simulink model "InvertedPendulumRobot_ControllerDesignLab"  (R2015b)
settings: Solver=FixedStepAuto  StartTime=0.0  StopTime=inf  RelTol=1e-3
libraries: arduinolib x10, simulink x2, aerolibtransform2 x1
settings Model: SimulationMode=external  ExtModeTrigDuration=2  Creator=james_000  LastModifiedBy=james_000
settings OptimizationCC: OptimizeModelRefInitCode=on  LifeSpan=1  MaxStackSize=64
settings DebuggingCC: InheritedTsInSrcMsg=none
settings HardwareCC: ProdBitPerInt=16  ProdBitPerPointer=16  ProdLargestAtomicFloat=None  ProdWordSize=8  ProdHWDeviceType=Atmel->AVR
settings RTWCC: SystemTargetFile=ert.tlc  TemplateMakefile=ert_default_tmf  Description=Embedded Coder  Toolchain=Arduino AVR v1.6.1  BuildConfiguration=Faster Runs  PortableWordSizes=on
settings CodeAppCC: IgnoreCustomStorageClasses=off
settings ERTTargetCC: SupportContinuousTime=on  SupportVariableSizeSignals=on  ExtMode=on  ExtModeMexArgs=0 7 115200

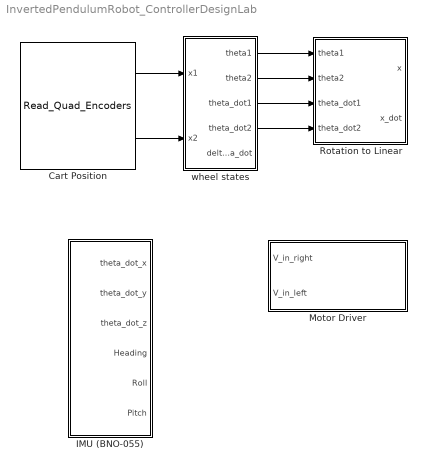
== system InvertedPendulumRobot_ControllerDesignLab ==
  Cart Position : S-Function  InitFcn=try, set_param(gcb,'FunctionName','Read_Quad_Encoders'), end  FunctionName=Read_Quad_Encoders  Parameters=uint8([0 1]),uint8([2 3]),uint8([7 8])  SFunctionModules=Read_Quad_Encoders_wrapper  SFunctionDeploymentMode=off  EnableBusSupport=off  mask(S-Function Builder){}
      mask help: Simulink:masks:SFunctionBuilder_MD
      mask init:
      | val = [[.9  0.75 0.75 1 1 .9 .9 1]',[1 1 0.75 0.75 .9 .9 1 .9]'];try , sys = get_param(gcb,'SfunBuilderFcnName');if isempty(sys), sys = get_param(gcb,'FunctionName'); end,catch, sys = get_param(gcb,'FunctionName'); end
      settings: CopyFcn=set_param(gcbh,'LinkStatus','none')  PreSaveFcn=try, set_param(gcb,'FunctionName','Read_Quad_Encoders'), end  OpenFcn=sfunctionwizard(gcbh)
      mask Display: plot(val(:,1),val(:,2)),disp(sys), port_label('output',1,'x1'), port_label('output',2,'x2')
  IMU (BNO-055) : Subsystem
  Motor Driver : Subsystem
  Rotation to Linear : Subsystem
  wheel states : Subsystem
  wires:
  Cart Position/1 -> wheel states/1(x1)
  Cart Position/2 -> wheel states/2(x2)
  wheel states/4(theta_dot2) -> Rotation to Linear/4(theta_dot2)
  wheel states/3(theta_dot1) -> Rotation to Linear/3(theta_dot1)
  wheel states/2(theta2) -> Rotation to Linear/2(theta2)
  wheel states/1(theta1) -> Rotation to Linear/1(theta1)

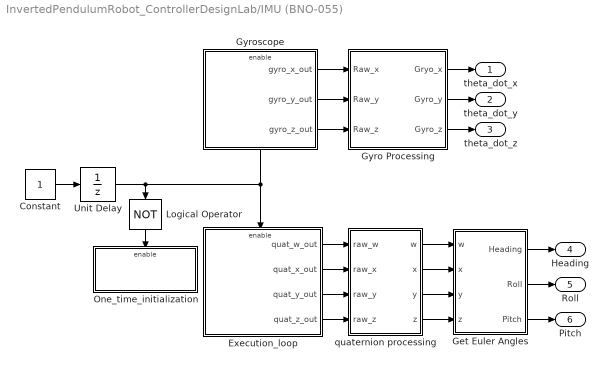
== system InvertedPendulumRobot_ControllerDesignLab/IMU (BNO-055) ==
  Constant : Constant  OutDataTypeStr=boolean  SampleTime=0.02
  Execution_loop : Subsystem  TreatAsAtomicUnit=on
  Get Euler Angles : Subsystem
  Gyro Processing : Subsystem
  Gyroscope : Subsystem  TreatAsAtomicUnit=on
  Logical Operator : Logic  Operator=NOT  AllPortsSameDT=off  OutDataTypeStr=boolean
  One_time_initialization : Subsystem  TreatAsAtomicUnit=on
  Unit Delay : UnitDelay  SampleTime=0.02
  quaternion processing : Subsystem
  theta_dot_x : Outport
  theta_dot_y : Outport  Port=2
  theta_dot_z : Outport  Port=3
  Heading : Outport  Port=4
  Roll : Outport  Port=5
  Pitch : Outport  Port=6
  wires:
  Constant/1 -> Unit Delay/1
  Logical Operator/1 -> One_time_initialization/Enable
  Unit Delay/1 -> Gyroscope/Enable, Execution_loop/Enable, Logical Operator/1
  Gyroscope/1(gyro_x_out) -> Gyro Processing/1(Raw_x)
  Gyroscope/2(gyro_y_out) -> Gyro Processing/2(Raw_y)
  Gyroscope/3(gyro_z_out) -> Gyro Processing/3(Raw_z)
  Gyro Processing/1(Gryo_x) -> theta_dot_x/1
  Gyro Processing/2(Gyro_y) -> theta_dot_y/1
  Gyro Processing/3(Gyro_z) -> theta_dot_z/1
  Get Euler Angles/1(Heading) -> Heading/1
  Execution_loop/1(quat_w_out) -> quaternion processing/1(raw_w)
  Execution_loop/2(quat_x_out) -> quaternion processing/2(raw_x)
  Execution_loop/3(quat_y_out) -> quaternion processing/3(raw_y)
  Execution_loop/4(quat_z_out) -> quaternion processing/4(raw_z)
  quaternion processing/1(w) -> Get Euler Angles/1(w)
  quaternion processing/2(x) -> Get Euler Angles/2(x)
  quaternion processing/3(y) -> Get Euler Angles/3(y)
  quaternion processing/4(z) -> Get Euler Angles/4(z)
  Get Euler Angles/2(Roll) -> Roll/1
  Get Euler Angles/3(Pitch) -> Pitch/1

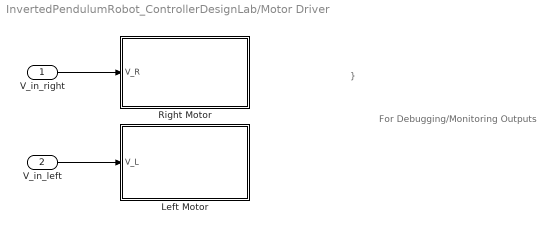
== system InvertedPendulumRobot_ControllerDesignLab/Motor Driver ==
  note: }
  note: For Debugging/Monitoring Outputs
  V_in_right : Inport
  V_in_left : Inport  Port=2
  Left Motor : Subsystem
  Right Motor : Subsystem
  wires:
  V_in_left/1 -> Left Motor/1(V_L)
  V_in_right/1 -> Right Motor/1(V_R)

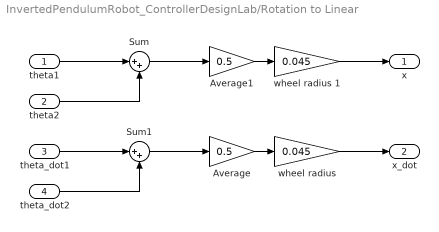
== system InvertedPendulumRobot_ControllerDesignLab/Rotation to Linear ==
  theta1 : Inport
  theta2 : Inport  Port=2
  theta_dot1 : Inport  Port=3
  theta_dot2 : Inport  Port=4
  Average : Gain  Gain=0.5
  Average1 : Gain  Gain=0.5
  Sum : Sum  Inputs=|++
  Sum1 : Sum  Inputs=|++
  wheel radius : Gain  Gain=0.045
  wheel radius 1 : Gain  Gain=0.045
  x : Outport
  x_dot : Outport  Port=2
  wires:
  theta2/1 -> Sum/2
  theta1/1 -> Sum/1
  Sum/1 -> Average1/1
  Average1/1 -> wheel radius 1/1
  theta_dot2/1 -> Sum1/2
  theta_dot1/1 -> Sum1/1
  Sum1/1 -> Average/1
  Average/1 -> wheel radius/1
  wheel radius 1/1 -> x/1
  wheel radius/1 -> x_dot/1

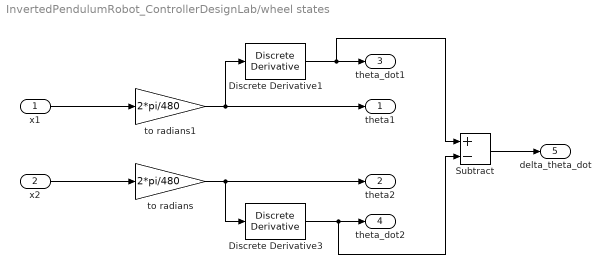
== system InvertedPendulumRobot_ControllerDesignLab/wheel states ==
  x1 : Inport
  x2 : Inport  Port=2
  Discrete Derivative1 : simulink/Discrete/Discrete Derivative  gainval=1.0  ICPrevScaledInput=0.0  InputProcessing=Inherited  OutMin=[]  OutMax=[]  OutDataType=fixdt(1, 16)  OutScaling=2^-10  DoSatur=off
  Discrete Derivative3 : simulink/Discrete/Discrete Derivative  gainval=1.0  ICPrevScaledInput=0.0  InputProcessing=Inherited  OutMin=[]  OutMax=[]  OutDataType=fixdt(1, 16)  OutScaling=2^-10  DoSatur=off
  Subtract : Sum  Inputs=+-
  to radians : Gain  Gain=2*pi/480
  to radians1 : Gain  Gain=2*pi/480
  theta1 : Outport
  theta2 : Outport  Port=2
  theta_dot1 : Outport  Port=3
  theta_dot2 : Outport  Port=4
  delta_theta_dot : Outport  Port=5
  wires:
  x2/1 -> to radians/1
  x1/1 -> to radians1/1
  to radians1/1 -> Discrete Derivative1/1, theta1/1
  Discrete Derivative1/1 -> Subtract/1, theta_dot1/1
  to radians/1 -> Discrete Derivative3/1, theta2/1
  Discrete Derivative3/1 -> Subtract/2, theta_dot2/1
  Subtract/1 -> delta_theta_dot/1

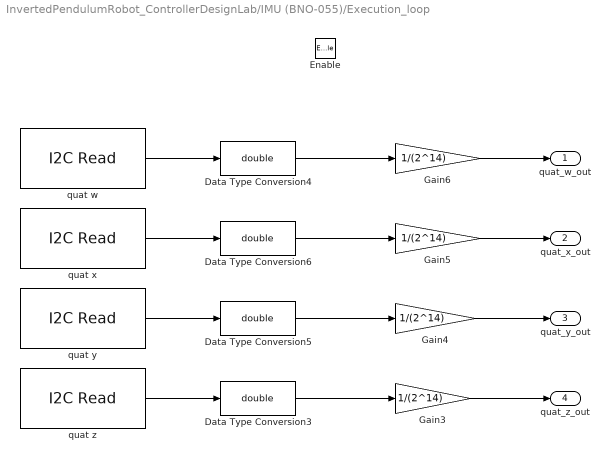
== system InvertedPendulumRobot_ControllerDesignLab/IMU (BNO-055)/Execution_loop ==
  Enable : EnablePort
  Data Type Conversion{3..6} (4 alike) : DataTypeConversion  OutDataTypeStr=double  ConvertRealWorld=Stored Integer (SI)
  Gain{3..6} (4 alike) : Gain  Gain=1/(2^14)
  quat w : arduinolib/I2C Read  SlaveAddress_=hex2dec( '28' )  RegisterAddressEnable=on  RegisterAddress_=hex2dec( '20' )  Datatype=uint16  ByteOrder=Little Endian  Datalength_=1  SampleTime_=0.02  blockPlatform=arduino
  quat x : arduinolib/I2C Read  SlaveAddress_=hex2dec( '28' )  RegisterAddressEnable=on  RegisterAddress_=hex2dec( '22' )  Datatype=uint16  ByteOrder=Little Endian  Datalength_=1  SampleTime_=0.02  blockPlatform=arduino
  quat y : arduinolib/I2C Read  SlaveAddress_=hex2dec( '28' )  RegisterAddressEnable=on  RegisterAddress_=hex2dec( '24' )  Datatype=uint16  ByteOrder=Little Endian  Datalength_=1  SampleTime_=0.02  blockPlatform=arduino
  quat z : arduinolib/I2C Read  SlaveAddress_=hex2dec( '28' )  RegisterAddressEnable=on  RegisterAddress_=hex2dec( '26' )  Datatype=uint16  ByteOrder=Little Endian  Datalength_=1  SampleTime_=0.02  blockPlatform=arduino
  quat_w_out : Outport
  quat_x_out : Outport  Port=2
  quat_y_out : Outport  Port=3
  quat_z_out : Outport  Port=4
  wires:
  quat x/1 -> Data Type Conversion6/1
  quat w/1 -> Data Type Conversion4/1
  quat y/1 -> Data Type Conversion5/1
  quat z/1 -> Data Type Conversion3/1
  Data Type Conversion4/1 -> Gain6/1
  Data Type Conversion6/1 -> Gain5/1
  Data Type Conversion5/1 -> Gain4/1
  Data Type Conversion3/1 -> Gain3/1
  Gain6/1 -> quat_w_out/1
  Gain5/1 -> quat_x_out/1
  Gain4/1 -> quat_y_out/1
  Gain3/1 -> quat_z_out/1

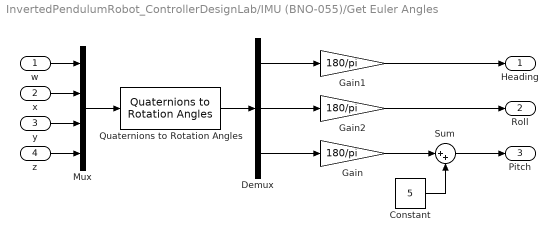
== system InvertedPendulumRobot_ControllerDesignLab/IMU (BNO-055)/Get Euler Angles ==
  w : Inport
  x : Inport  Port=2
  y : Inport  Port=3
  z : Inport  Port=4
  Constant : Constant  Value=5
  Demux : Demux  Outputs=3
  Gain : Gain  Gain=180/pi
  Gain1 : Gain  Gain=180/pi
  Gain2 : Gain  Gain=180/pi
  Mux : Mux
  Quaternions to Rotation Angles : aerolibtransform2/Quaternions to Rotation Angles  rotationOrder=ZYX
  Sum : Sum  Inputs=|++
  Heading : Outport
  Roll : Outport  Port=2
  Pitch : Outport  Port=3
  wires:
  Mux/1 -> Quaternions to Rotation Angles/1
  Quaternions to Rotation Angles/1 -> Demux/1
  Demux/2 -> Gain2/1
  Demux/1 -> Gain1/1
  w/1 -> Mux/1
  x/1 -> Mux/2
  y/1 -> Mux/3
  z/1 -> Mux/4
  Demux/3 -> Gain/1
  Sum/1 -> Pitch/1
  Constant/1 -> Sum/2
  Gain/1 -> Sum/1
  Gain2/1 -> Roll/1
  Gain1/1 -> Heading/1

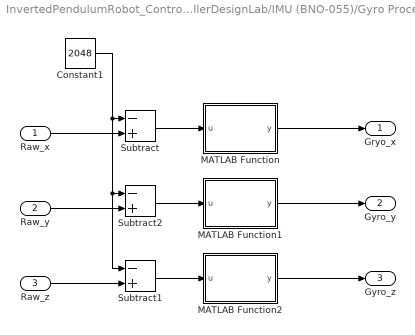
== system InvertedPendulumRobot_ControllerDesignLab/IMU (BNO-055)/Gyro Processing ==
  Raw_x : Inport
  Raw_y : Inport  Port=2
  Raw_z : Inport  Port=3
  Constant1 : Constant  Value=2048  OutDataTypeStr=double
  MATLAB Function : MATLAB Function  TreatAsAtomicUnit=on
  MATLAB Function1 : MATLAB Function  TreatAsAtomicUnit=on
  MATLAB Function2 : MATLAB Function  TreatAsAtomicUnit=on
  Subtract : Sum  Inputs=-+  OutDataTypeStr=double
  Subtract1 : Sum  Inputs=-+  OutDataTypeStr=double
  Subtract2 : Sum  Inputs=-+  OutDataTypeStr=double
  Gryo_x : Outport
  Gyro_y : Outport  Port=2
  Gyro_z : Outport  Port=3
  wires:
  Raw_x/1 -> Subtract/2
  Raw_z/1 -> Subtract1/2
  Raw_y/1 -> Subtract2/2
  MATLAB Function1/1(y) -> Gyro_y/1
  Subtract/1 -> MATLAB Function/1(u)
  Subtract2/1 -> MATLAB Function1/1(u)
  Subtract1/1 -> MATLAB Function2/1(u)
  Constant1/1 -> Subtract/1, Subtract2/1, Subtract1/1
  MATLAB Function/1(y) -> Gryo_x/1
  MATLAB Function2/1(y) -> Gyro_z/1

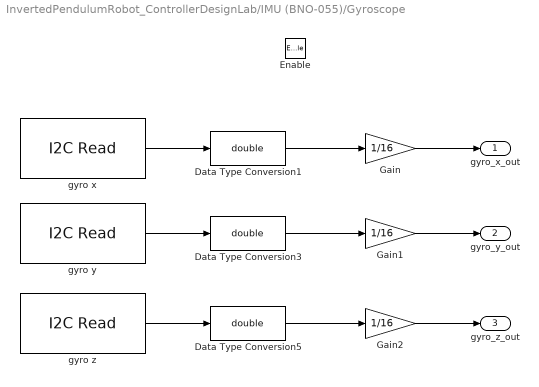
== system InvertedPendulumRobot_ControllerDesignLab/IMU (BNO-055)/Gyroscope ==
  Enable : EnablePort
  Data Type Conversion1 : DataTypeConversion  OutDataTypeStr=double
  Data Type Conversion3 : DataTypeConversion  OutDataTypeStr=double
  Data Type Conversion5 : DataTypeConversion  OutDataTypeStr=double
  Gain : Gain  Gain=1/16  OutDataTypeStr=Inherit: Same as input
  Gain1 : Gain  Gain=1/16  OutDataTypeStr=Inherit: Same as input
  Gain2 : Gain  Gain=1/16  OutDataTypeStr=Inherit: Same as input
  gyro x : arduinolib/I2C Read  SlaveAddress_=hex2dec( '28' )  RegisterAddressEnable=on  RegisterAddress_=hex2dec( '14' )  Datatype=uint16  ByteOrder=Little Endian  Datalength_=1  SampleTime_=0.02  blockPlatform=arduino
  gyro y : arduinolib/I2C Read  SlaveAddress_=hex2dec( '28' )  RegisterAddressEnable=on  RegisterAddress_=hex2dec( '16' )  Datatype=uint16  ByteOrder=Little Endian  Datalength_=1  SampleTime_=0.02  blockPlatform=arduino
  gyro z : arduinolib/I2C Read  SlaveAddress_=hex2dec( '28' )  RegisterAddressEnable=on  RegisterAddress_=hex2dec( '18' )  Datatype=uint16  ByteOrder=Little Endian  Datalength_=1  SampleTime_=0.02  blockPlatform=arduino
  gyro_x_out : Outport
  gyro_y_out : Outport  Port=2
  gyro_z_out : Outport  Port=3
  wires:
  Gain/1 -> gyro_x_out/1
  Gain1/1 -> gyro_y_out/1
  Gain2/1 -> gyro_z_out/1
  gyro x/1 -> Data Type Conversion1/1
  Data Type Conversion3/1 -> Gain1/1
  Data Type Conversion5/1 -> Gain2/1
  gyro y/1 -> Data Type Conversion3/1
  gyro z/1 -> Data Type Conversion5/1
  Data Type Conversion1/1 -> Gain/1

== system InvertedPendulumRobot_ControllerDesignLab/IMU (BNO-055)/One_time_initialization ==
  Enable : EnablePort
  Constant2 : Constant  Value=8  OutDataTypeStr=uint8
  I2C Write2 : arduinolib/I2C Write  Priority=1  SlaveAddress_=hex2dec( '28' )  RegisterAddressEnable=on  RegisterAddress_=hex2dec( '3D' )  Datatype=uint8  ByteOrder=Big Endian  blockPlatform=arduino
      settings: AttributesFormatString=Priority=%<Priority>
  wires:
  Constant2/1 -> I2C Write2/1

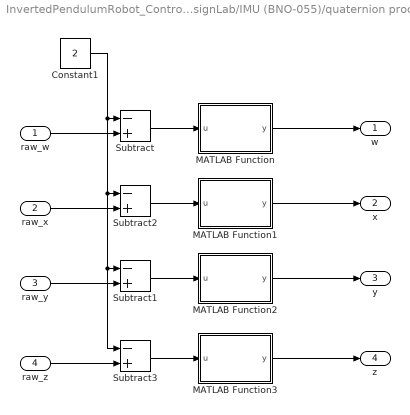
== system InvertedPendulumRobot_ControllerDesignLab/IMU (BNO-055)/quaternion processing ==
  raw_w : Inport
  raw_x : Inport  Port=2
  raw_y : Inport  Port=3
  raw_z : Inport  Port=4
  Constant1 : Constant  Value=2  OutDataTypeStr=double
  MATLAB Function : MATLAB Function  TreatAsAtomicUnit=on
  MATLAB Function1 : MATLAB Function  TreatAsAtomicUnit=on
  MATLAB Function2 : MATLAB Function  TreatAsAtomicUnit=on
  MATLAB Function3 : MATLAB Function  TreatAsAtomicUnit=on
  Subtract{,1..3} (4 alike) : Sum  Inputs=-+  OutDataTypeStr=double
  w : Outport
  x : Outport  Port=2
  y : Outport  Port=3
  z : Outport  Port=4
  wires:
  raw_x/1 -> Subtract2/2
  Subtract2/1 -> MATLAB Function1/1(u)
  Subtract1/1 -> MATLAB Function2/1(u)
  Subtract/1 -> MATLAB Function/1(u)
  raw_w/1 -> Subtract/2
  raw_y/1 -> Subtract1/2
  MATLAB Function1/1(y) -> x/1
  Constant1/1 -> Subtract/1, Subtract2/1, Subtract3/1, Subtract1/1
  MATLAB Function2/1(y) -> y/1
  MATLAB Function/1(y) -> w/1
  Subtract3/1 -> MATLAB Function3/1(u)
  raw_z/1 -> Subtract3/2
  MATLAB Function3/1(y) -> z/1

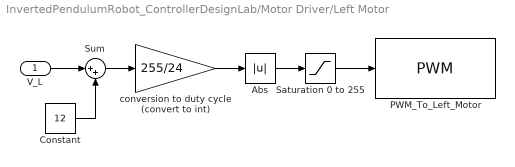
== system InvertedPendulumRobot_ControllerDesignLab/Motor Driver/Left Motor ==
  V_L : Inport
  Abs : Abs
  Constant : Constant  Value=12
  PWM_To_Left_Motor : arduinolib/PWM  pinNumber=5  blockPlatform=arduino
  Saturation 0 to 255 : Saturate  UpperLimit=255  LowerLimit=0
  Sum : Sum  Inputs=|++
  conversion to duty cycle (convert to int) : Gain  Gain=255/24  OutDataTypeStr=int16
  wires:
  Saturation 0 to 255/1 -> PWM_To_Left_Motor/1
  conversion to duty cycle (convert to int)/1 -> Abs/1
  Abs/1 -> Saturation 0 to 255/1
  V_L/1 -> Sum/1
  Sum/1 -> conversion to duty cycle (convert to int)/1
  Constant/1 -> Sum/2

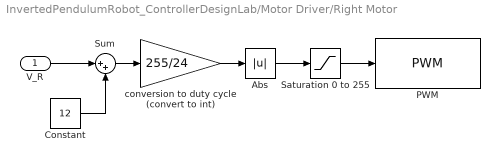
== system InvertedPendulumRobot_ControllerDesignLab/Motor Driver/Right Motor ==
  V_R : Inport
  Abs : Abs
  Constant : Constant  Value=12
  PWM : arduinolib/PWM  pinNumber=3  blockPlatform=arduino
  Saturation 0 to 255 : Saturate  UpperLimit=255  LowerLimit=0
  Sum : Sum  Inputs=|++
  conversion to duty cycle (convert to int) : Gain  Gain=255/24  OutDataTypeStr=int16
  wires:
  Abs/1 -> Saturation 0 to 255/1
  Saturation 0 to 255/1 -> PWM/1
  conversion to duty cycle (convert to int)/1 -> Abs/1
  V_R/1 -> Sum/1
  Sum/1 -> conversion to duty cycle (convert to int)/1
  Constant/1 -> Sum/2

== matlab function InvertedPendulumRobot_ControllerDesignLab/IMU (BNO-055)/Gyro Processing/MATLAB Function1 ==
  data: u input; y output
function y = fcn(u)
%#codegen
if u>1000
    u=u-2048;
elseif u<1000
    u=u+2048;
else
    u=u;
end
y = u;

== matlab function InvertedPendulumRobot_ControllerDesignLab/IMU (BNO-055)/Gyro Processing/MATLAB Function ==
  data: u input; y output
function y = fcn(u)
%#codegen
if u>1000
    u=u-2048;
elseif u<1000
    u=u+2048;
else
    u=u;
end
y = u;

== matlab function InvertedPendulumRobot_ControllerDesignLab/IMU (BNO-055)/Gyro Processing/MATLAB Function2 ==
  data: u input; y output
function y = fcn(u)
%#codegen
if u>1000
    u=u-2048;
elseif u<1000
    u=u+2048;
else
    u=u;
end
y = u;

== matlab function InvertedPendulumRobot_ControllerDesignLab/IMU (BNO-055)/quaternion processing/MATLAB Function ==
  data: u input; y output
function y = fcn(u)
%#codegen
if u>1
    u=u-2;
elseif u<-1
    u=u+2;
end
y = u;

== matlab function InvertedPendulumRobot_ControllerDesignLab/IMU (BNO-055)/quaternion processing/MATLAB Function1 ==
  data: u input; y output
function y = fcn(u)
%#codegen
if u>1
    u=u-2;
elseif u<-1
    u=u+2;
end
y = u;

== matlab function InvertedPendulumRobot_ControllerDesignLab/IMU (BNO-055)/quaternion processing/MATLAB Function2 ==
  data: u input; y output
function y = fcn(u)
%#codegen
if u>1
    u=u-2;
elseif u<-1
    u=u+2;
end
y = u;

== matlab function InvertedPendulumRobot_ControllerDesignLab/IMU (BNO-055)/quaternion processing/MATLAB Function3 ==
  data: u input; y output
function y = fcn(u)
%#codegen
if u>1
    u=u-2;
elseif u<-1
    u=u+2;
end
y = u;
